simulink library "real_comp_2c4t_lib"  (Simulink 8.7)
settings: Solver=ode45  StartTime=0.0  StopTime=10.0  RelTol=1e-3
undefined symbols (not defined in the file): AdvDSPBChannelOutDisplay, dpoly, dspba_ChannelInVis, dspba_ChannelOutVis, dspba_internal_get_channel_ports, dspba_internal_get_demux_ports, evalAionMaskParam, latency, primtype, value
libraries: DSPBAPrim x17, Pipereg_lib x2, DSPBABase x1
settings Model: Creator=bigcat  LastModifiedBy=5g

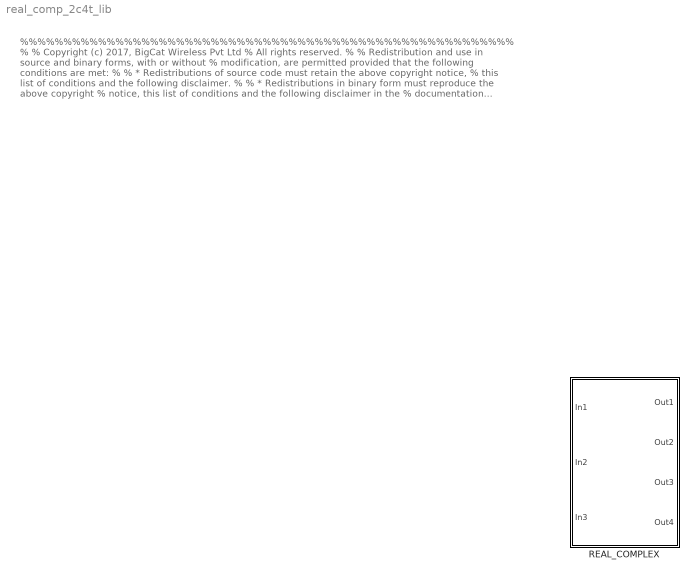
== system real_comp_2c4t_lib ==
  note: %%%%%%%%%%%%%%%%%%%%%%%%%%%%%%%%%%%%%%%%%%%%%%%%%%%%%%%%%
      |  %
      |  % Copyright (c) 2017, BigCat Wireless Pvt Ltd
      |  % All rights reserved.
      |  %
      |  % Redistribution and use in source and binary forms, with or without
      |  % modification, are permitted provided that the following conditions are met:
      |  %
      |  %     * Redistributions of source code must retain the above copyright notice,
      |  %       this list of conditions and the following disclaimer.
      |  %
      |  %     * Redistributions in binary form must reproduce the above copyright
      |  %       notice, this list of conditions and the following disclaimer in the
      |  %       documentation and/or other materials provided with the distribution.
      |  %
      |  %     * Neither the name of the copyright holder nor the names of its contributors
      |  %       may be used to endorse or promote products derived from this software
      |  %       without specific prior written permission.
      |  %
      |  %
      |  %
      |  % THIS SOFTWARE IS PROVIDED BY THE COPYRIGHT HOLDERS AND CONTRIBUTORS "AS IS"
      |  % AND ANY EXPRESS OR IMPLIED WARRANTIES, INCLUDING, BUT NOT LIMITED TO, THE
      |  % IMPLIED WARRANTIES OF MERCHANTABILITY AND FITNESS FOR A PARTICULAR PURPOSE ARE
      |  % DISCLAIMED. IN NO EVENT SHALL THE COPYRIGHT HOLDER OR CONTRIBUTORS BE LIABLE
      |  % FOR ANY DIRECT, INDIRECT, INCIDENTAL, SPECIAL, EXEMPLARY, OR CONSEQUENTIAL
      |  % DAMAGES (INCLUDING, BUT NOT LIMITED TO, PROCUREMENT OF SUBSTITUTE GOODS OR
      |  % SERVICES; LOSS OF USE, DATA, OR PROFITS; OR BUSINESS INTERRUPTION) HOWEVER
      |  % CAUSED AND ON ANY THEORY OF LIABILITY, WHETHER IN CONTRACT, STRICT LIABILITY,
      |  % OR TORT (INCLUDING NEGLIGENCE OR OTHERWISE) ARISING IN ANY WAY OUT OF THE USE
      |  % OF THIS SOFTWARE, EVEN IF ADVISED OF THE POSSIBILITY OF SUCH DAMAGE.
      |  %
      |   %%%%%%%%%%%%%%%%%%%%%%%%%%%%%%%%%%%%%%%%%%%%%%%%%%%%%%%%%%
  "REAL_COMPLEX " : Subsystem  mask{ClockMargin=0, Latency=0, Pipeline_stages=0}
      mask Display:
      | disp('REAL_COMPLEX');
      | port_label('input',2,'v');
      | port_label('input',3,'c');
      | port_label('input',1,'d');
      | port_label('output',3,'q_v');
      | port_label('output',4,'q_c');
      | port_label('output',1,'q0');
      | port_label('output',2,'q1');

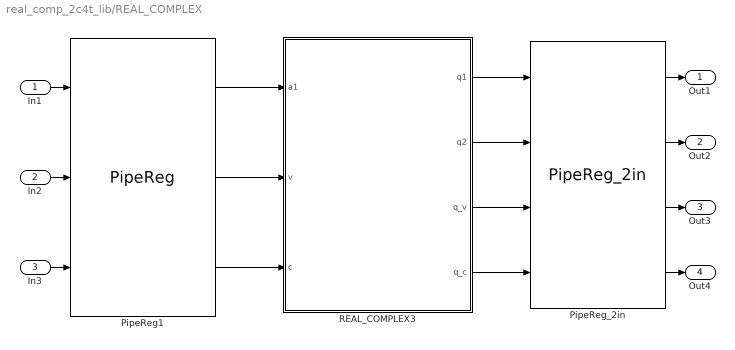
== system real_comp_2c4t_lib/REAL_COMPLEX  ==
  In1 : Inport
  In2 : Inport  Port=2
  In3 : Inport  Port=3
  PipeReg1 : Pipereg_lib/PipeReg  NPipe=Pipeline_stages  Clock_Margin=ClockMargin
  PipeReg_2in : Pipereg_lib/PipeReg_2in  NPipe=Pipeline_stages  Clock_Margin=ClockMargin
  REAL_COMPLEX3 : Subsystem
  Out1 : Outport
  Out2 : Outport  Port=2
  Out3 : Outport  Port=3
  Out4 : Outport  Port=4
  wires:
  In1/1 -> PipeReg1/1
  PipeReg1/2 -> REAL_COMPLEX3/2(v)
  PipeReg1/3 -> REAL_COMPLEX3/3(c)
  REAL_COMPLEX3/3(q_v) -> PipeReg_2in/3
  In2/1 -> PipeReg1/2
  PipeReg_2in/1 -> Out1/1
  REAL_COMPLEX3/2(q2) -> PipeReg_2in/2
  REAL_COMPLEX3/4(q_c) -> PipeReg_2in/4
  PipeReg1/1 -> REAL_COMPLEX3/1(a1)
  PipeReg_2in/3 -> Out3/1
  PipeReg_2in/4 -> Out4/1
  In3/1 -> PipeReg1/3
  PipeReg_2in/2 -> Out2/1
  REAL_COMPLEX3/1(q1) -> PipeReg_2in/1

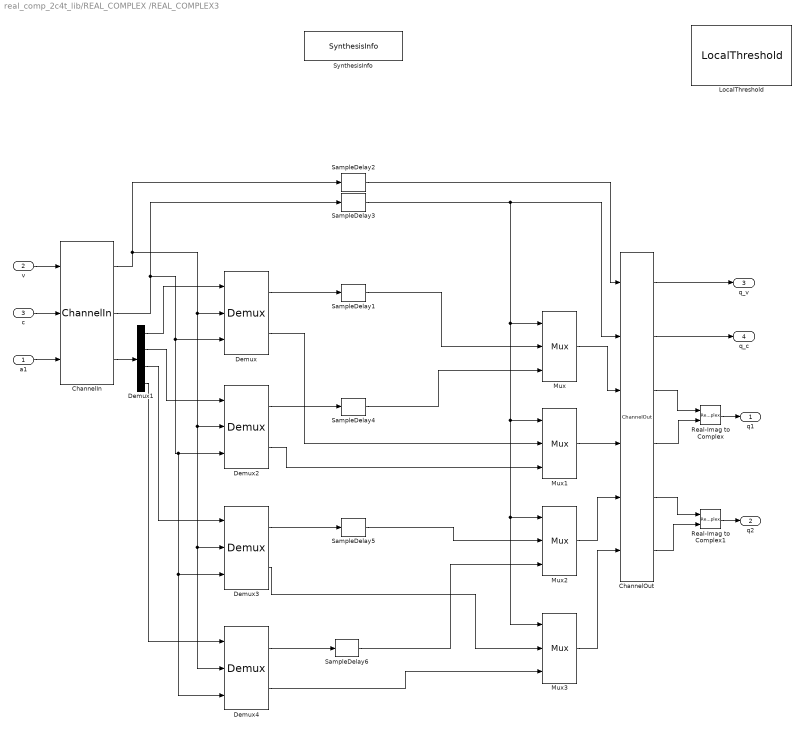
== system real_comp_2c4t_lib/REAL_COMPLEX /REAL_COMPLEX3 ==
  a1 : Inport
  v : Inport  Port=2
  c : Inport  Port=3
  ChannelIn : DSPBAPrim/ChannelIn  primtype=channelin  nInputs=dspba_internal_get_channel_ports(gcb)  nOutputs=dspba_internal_get_channel_ports(gcb)  omode=Inherit via internal rule  otype=sfix(16)  scale=2^-15  rndmethod=Unbiased  factor=1  satmethod=Symmetric  shift_vec=[0 1 2 -1]  value=1  inPortNames=['v'; 'c'; '0'; '1'; '2'; '3'; '4'; '5'; '6'; '7'; '8'; '9'; 'A'; 'B'; 'D'; 'E'; 'F'; 'G'; 'H'; 'I'; 'J'; 'K'; 'L'; 'M'; 'N'; 'O'; 'P'; 'Q'; 'R'; 'S'; 'T'; 'U'; 'W'; 'X'; 'Y'; 'Z']  outPortNames=['v'; 'c'; '0'; '1'; '2'; '3'; '4'; '5'; '6'; '7'; '8'; '9'; 'A'; 'B'; 'D'; 'E'; 'F'; 'G'; 'H'; 'I'; 'J'; 'K'; 'L'; 'M'; 'N'; 'O'; 'P'; 'Q'; 'R'; 'S'; 'T'; 'U'; 'W'; 'X'; 'Y'; 'Z']  dspbaimage=dspba_prim.jpg  text=fprintf('In');  style=Optimised  dataSignals=1  foldingEnabled=off  channels=1  sampleRate=200  packetBeginPresent=off  packetBeginEnabled=off  visibilities=dspba_ChannelInVis(gcb)  latencyCorrection=0  version=20141013
  ChannelOut : DSPBAPrim/ChannelOut  primtype=channelout  nInputs=dspba_internal_get_channel_ports(gcb)  nOutputs=dspba_internal_get_channel_ports(gcb)  omode=Inherit via internal rule  otype=sfix(16)  scale=2^-15  rndmethod=Unbiased  factor=1  satmethod=Symmetric  shift_vec=[0 1 2 -1]  value=4  inPortNames=['v'; 'c'; '0'; '1'; '2'; '3'; '4'; '5'; '6'; '7'; '8'; '9'; 'A'; 'B'; 'D'; 'E'; 'F'; 'G'; 'H'; 'I'; 'J'; 'K'; 'L'; 'M'; 'N'; 'O'; 'P'; 'Q'; 'R'; 'S'; 'T'; 'U'; 'W'; 'X'; 'Y'; 'Z']  outPortNames=['v'; 'c'; '0'; '1'; '2'; '3'; '4'; '5'; '6'; '7'; '8'; '9'; 'A'; 'B'; 'D'; 'E'; 'F'; 'G'; 'H'; 'I'; 'J'; 'K'; 'L'; 'M'; 'N'; 'O'; 'P'; 'Q'; 'R'; 'S'; 'T'; 'U'; 'W'; 'X'; 'Y'; 'Z']  dspbaimage=dspba_prim.jpg  text=fprintf('Out%s', AdvDSPBChannelOutDisplay(latency));  style=Optimised  dataSignals=4  foldingEnabled=off  channels=1  sampleRate=200  packetBeginPresent=off  packetBeginEnabled=off  visibilities=dspba_ChannelOutVis(gcb)  latency=21  latencyCorrection=0  version=20141013
  Demux{,2..4} (4 alike) : DSPBAPrim/Demux  primtype=demux  nInputs=3  nOutputs=dspba_internal_get_demux_ports(gcb)  omode=Inherit via internal rule  otype=sfix(16)  scale=2^-15  rndmethod=Unbiased  factor=1  satmethod=Symmetric  shift_vec=[0 1]  value=2  inPortNames=['q'; 'v'; 'c']  outPortNames=['c0'; 'c1']  dspbaimage=dspba_prim.jpg  text=fprintf('demux');  style=Optimised  visibilities=1536  version=20100120
  Demux1 : Demux
  LocalThreshold : DSPBABase/LocalThreshold  margin=ClockMargin  delayRegOrRAMThresholdBits=10000  MediumDualMemThresholdBits=10000  LargeDualMemThresholdBits=-1  hardMultiplierThresholdLuts=-1  version=0
  Mux{,1..3} (4 alike) : DSPBAPrim/Mux  primtype=mux  nInputs=evalAionMaskParam(gcb,'value',1)+1  nOutputs=1  omode=Inherit via internal rule  otype=sfix(16)  scale=2^-15  rndmethod=Unbiased  factor=1  satmethod=Symmetric  shift_vec=[0 1 2 -1]  value=2  inPortNames=['s '; 'd0'; 'd1'; 'd2'; 'd3'; 'd4'; 'd5'; 'd6'; 'd7'; 'd8'; 'd9';]  outPortNames=[' ']  dspbaimage=dspba_prim.jpg  text=fprintf('%s', primtype);  style=Optimised  visibilities=1032  version=20131025
  Real-Imag to Complex : RealImagToComplex
  Real-Imag to Complex1 : RealImagToComplex
  SampleDelay{1..6} (6 alike) : DSPBAPrim/SampleDelay  primtype=sampdelay  nInputs=1  nOutputs=1  omode=Inherit via internal rule  otype=sfix(16)  scale=2^-15  rndmethod=Unbiased  factor=1  satmethod=Symmetric  shift_vec=[0 1 2 -1]  value=1  inPortNames=[' '; ' ';]  outPortNames=[' ']  dspbaimage=dspba_prim.jpg  text=dpoly(1, eye(1,value+1), 'z')  style=Optimised  visibilities=8 + 1024 + 2^17 + 2^18  flexible=off  slackgroup=0  augmented=0  version=20090407  advOptions=[]
  SynthesisInfo : DSPBAPrim/SynthesisInfo  primtype=synthinfo  nInputs=0  nOutputs=0  omode=Inherit via internal rule  otype=sfix(16)  scale=2^-15  rndmethod=Truncate  factor=1  satmethod=Symmetric  shift_vec=[0 1 2 -1]  value=99  inPortNames=[' '; ' ';]  outPortNames=[' ']  dspbaimage=dspba_prim_ctrl.jpg  text=fprintf('Style=%s', style);  style=Scheduled  visibilities=2^15+2^17+2^18+2^19  constraintInUse=on  constraintRelation=>  constraintLimit=Latency  bitAccurate=off  version=20090407
  q1 : Outport
  q2 : Outport  Port=2
  q_v : Outport  Port=3
  q_c : Outport  Port=4
  wires:
  SampleDelay4/1 -> Mux/3
  SampleDelay1/1 -> Mux/2
  ChannelIn/1 -> Demux3/2, Demux4/2, Demux2/2, Demux/2, SampleDelay2/1
  Real-Imag to Complex/1 -> q1/1
  ChannelOut/4 -> Real-Imag to Complex/2
  Demux/1 -> SampleDelay1/1
  ChannelOut/2 -> q_c/1
  ChannelIn/2 -> Demux3/3, Demux4/3, Demux2/3, Demux/3, SampleDelay3/1
  Mux1/1 -> ChannelOut/4
  Mux/1 -> ChannelOut/3
  ChannelOut/3 -> Real-Imag to Complex/1
  ChannelOut/1 -> q_v/1
  c/1 -> ChannelIn/2
  v/1 -> ChannelIn/1
  a1/1 -> ChannelIn/3
  ChannelIn/3 -> Demux1/1
  Demux1/1 -> Demux/1
  Demux1/2 -> Demux2/1
  Demux2/1 -> SampleDelay4/1
  Demux/2 -> Mux1/2
  Demux2/2 -> Mux1/3
  SampleDelay2/1 -> ChannelOut/1
  SampleDelay3/1 -> ChannelOut/2, Mux2/1, Mux3/1, Mux1/1, Mux/1
  Demux1/3 -> Demux3/1
  Demux1/4 -> Demux4/1
  Mux2/1 -> ChannelOut/5
  Mux3/1 -> ChannelOut/6
  Demux3/1 -> SampleDelay5/1
  SampleDelay5/1 -> Mux2/2
  SampleDelay6/1 -> Mux2/3
  Demux4/1 -> SampleDelay6/1
  Demux3/2 -> Mux3/2
  Demux4/2 -> Mux3/3
  Real-Imag to Complex1/1 -> q2/1
  ChannelOut/5 -> Real-Imag to Complex1/1
  ChannelOut/6 -> Real-Imag to Complex1/2
